simulink model "PositionControl"  (R2020b)
settings: Solver=ode3  StartTime=0.0  StopTime=100.0  FixedStep=Ts  RelTol=1e-3
values from neighbouring files (symbols this model uses):
  refx = rand    [CompararResultados.m]    (also in RunPositionControl.m = (rand-rand)*10)
  refy = rand    [CompararResultados.m]    (also in RunPositionControl.m = (rand-rand)*10)
undefined symbols (not defined in the file or in its folder): DiscIntNeverNeededParam
libraries: simulink x1
settings Model: Creator=patri  LastModifiedBy=patri
settings DataIOCC: ReturnWorkspaceOutputs=off

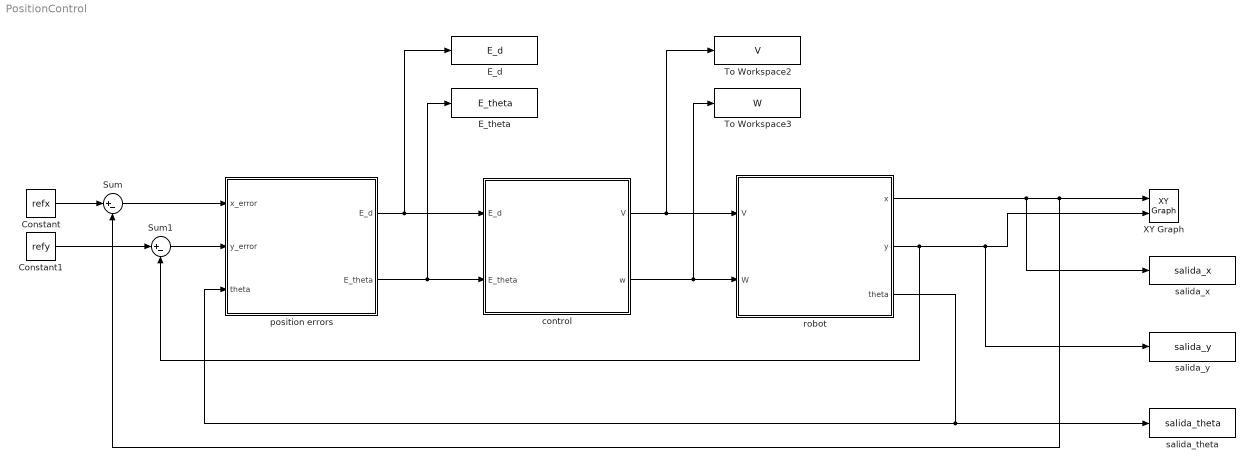
== system PositionControl ==
  Constant : Constant  Value=refx
  Constant1 : Constant  Value=refy
  E_d : ToWorkspace  VariableName=E_d  SaveFormat=Timeseries  SampleTime=-1
  E_theta : ToWorkspace  VariableName=E_theta  SaveFormat=Timeseries  SampleTime=-1
  Sum : Sum  Inputs=|+-
  Sum1 : Sum  Inputs=|+-
  To Workspace2 : ToWorkspace  VariableName=V  SaveFormat=Timeseries  SampleTime=-1
  To Workspace3 : ToWorkspace  VariableName=W  SaveFormat=Timeseries  SampleTime=-1
  XY Graph : simulink/Sinks/XY Graph  xmin=-5  xmax=5  ymin=-5  ymax=5  st=-1
  control : Subsystem
  position errors : Subsystem
  robot : Subsystem
  salida_theta : ToWorkspace  VariableName=salida_theta  SaveFormat=Timeseries  SampleTime=-1
  salida_x : ToWorkspace  VariableName=salida_x  SaveFormat=Timeseries  SampleTime=-1
  salida_y : ToWorkspace  VariableName=salida_y  SaveFormat=Timeseries  SampleTime=-1
  wires:
  control/1(V) -> robot/1(V), To Workspace2/1
  position errors/1("E_d ") -> control/1(E_d), E_d/1
  Sum1/1 -> position errors/2("y_error ")
  Sum/1 -> position errors/1("x_error ")
  Constant/1 -> Sum/1
  Constant1/1 -> Sum1/1
  robot/1("x ") -> salida_x/1, Sum/2, XY Graph/1
  control/2(w) -> robot/2("W "), To Workspace3/1
  robot/2(y) -> Sum1/2, salida_y/1, XY Graph/2
  robot/3(theta) -> salida_theta/1, position errors/3(theta)
  position errors/2(E_theta) -> E_theta/1, control/2(E_theta)

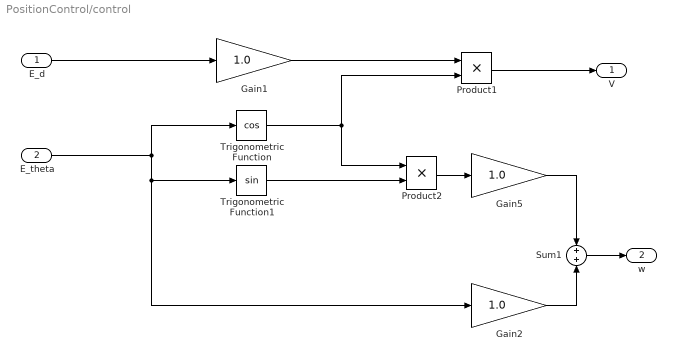
== system PositionControl/control ==
  E_d : Inport
  E_theta : Inport  Port=2
  Gain1 : Gain  Gain=1.0
  Gain2 : Gain  Gain=1.0
  Gain5 : Gain  Gain=1.0
  Product1 : Product
  Product2 : Product
  Sum1 : Sum
  Trigonometric Function : Trigonometry  Operator=cos
  Trigonometric Function1 : Trigonometry
  V : Outport  VectorParamsAs1DForOutWhenUnconnected=off
  w : Outport  Port=2  VectorParamsAs1DForOutWhenUnconnected=off
  wires:
  E_theta/1 -> Gain2/1, Trigonometric Function1/1, Trigonometric Function/1
  E_d/1 -> Gain1/1
  Trigonometric Function/1 -> Product1/2, Product2/1
  Product1/1 -> V/1
  Trigonometric Function1/1 -> Product2/2
  Product2/1 -> Gain5/1
  Gain1/1 -> Product1/1
  Gain5/1 -> Sum1/1
  Gain2/1 -> Sum1/2
  Sum1/1 -> w/1

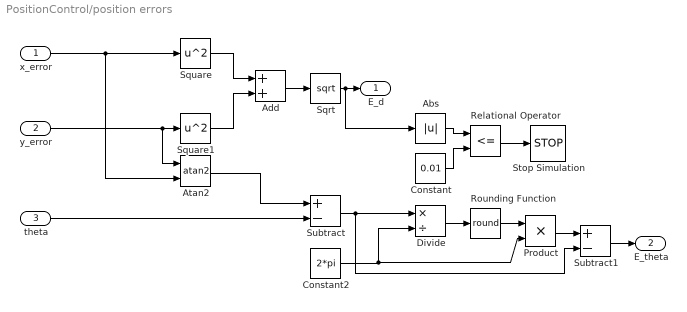
== system PositionControl/position errors ==
  "x_error " : Inport
  "y_error " : Inport  Port=2
  theta : Inport  Port=3
  Abs : Abs
  Add : Sum
  Atan2 : Trigonometry  Operator=atan2
  Constant : Constant  Value=0.01
  Constant2 : Constant  Value=2*pi
  Divide : Product  Inputs=*/
  Product : Product
  Relational Operator : RelationalOperator  Operator=<=  OutDataTypeStr=boolean  RndMeth=Simplest
  Rounding Function : Rounding  Operator=round
  Sqrt : Sqrt  SaturateOnIntegerOverflow=on
  Square : Math  Operator=square  SaturateOnIntegerOverflow=on
  Square1 : Math  Operator=square  SaturateOnIntegerOverflow=on
  Stop Simulation : Stop
  Subtract : Sum  Inputs=+-  OutMin=[-pi]  OutMax=[pi]
  Subtract1 : Sum  Inputs=+-  OutMin=[-pi]  OutMax=[pi]
  "E_d " : Outport
  E_theta : Outport  Port=2
  wires:
  Subtract1/1 -> E_theta/1
  Subtract/1 -> Subtract1/2, Divide/1
  Product/1 -> Subtract1/1
  Constant2/1 -> Product/2, Divide/2
  Square/1 -> Add/1
  "x_error "/1 -> Atan2/2, Square/1
  Abs/1 -> Relational Operator/1
  Rounding Function/1 -> Product/1
  Divide/1 -> Rounding Function/1
  Constant/1 -> Relational Operator/2
  Sqrt/1 -> Abs/1, "E_d "/1
  Square1/1 -> Add/2
  Add/1 -> Sqrt/1
  Relational Operator/1 -> Stop Simulation/1
  Atan2/1 -> Subtract/1
  "y_error "/1 -> Atan2/1, Square1/1
  theta/1 -> Subtract/2

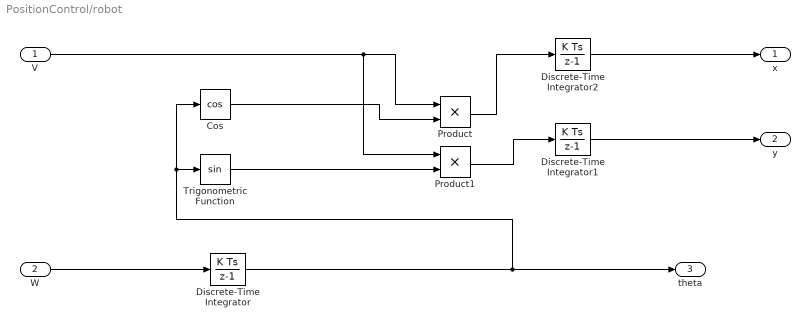
== system PositionControl/robot ==
  V : Inport
  "W " : Inport  Port=2
  Cos : Trigonometry  Operator=cos
  Discrete-Time Integrator : DiscreteIntegrator  SampleTime=-1  ICPrevOutput=DiscIntNeverNeededParam  ICPrevScaledInput=DiscIntNeverNeededParam
  Discrete-Time Integrator1 : DiscreteIntegrator  SampleTime=-1  ICPrevOutput=DiscIntNeverNeededParam  ICPrevScaledInput=DiscIntNeverNeededParam
  Discrete-Time Integrator2 : DiscreteIntegrator  SampleTime=-1  ICPrevOutput=DiscIntNeverNeededParam  ICPrevScaledInput=DiscIntNeverNeededParam
  Product : Product
  Product1 : Product
  Trigonometric Function : Trigonometry
  "x " : Outport
  y : Outport  Port=2
  theta : Outport  Port=3
  wires:
  Discrete-Time Integrator1/1 -> y/1
  "W "/1 -> Discrete-Time Integrator/1
  Trigonometric Function/1 -> Product1/2
  Product1/1 -> Discrete-Time Integrator1/1
  Discrete-Time Integrator2/1 -> "x "/1
  Product/1 -> Discrete-Time Integrator2/1
  Cos/1 -> Product/2
  V/1 -> Product1/1, Product/1
  Discrete-Time Integrator/1 -> theta/1, Cos/1, Trigonometric Function/1
